simulink model "randomStuff"  (R2025a)
settings: Solver=VariableStepAuto  StartTime=0.0  StopTime=10.0  RelTol=1e-3
settings Model: Creator=willager  LastModifiedBy=willager

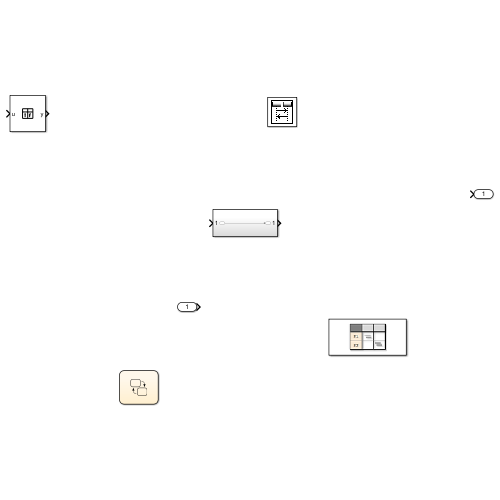
[thumbnail: Simulink's stored preview of the top-level diagram]
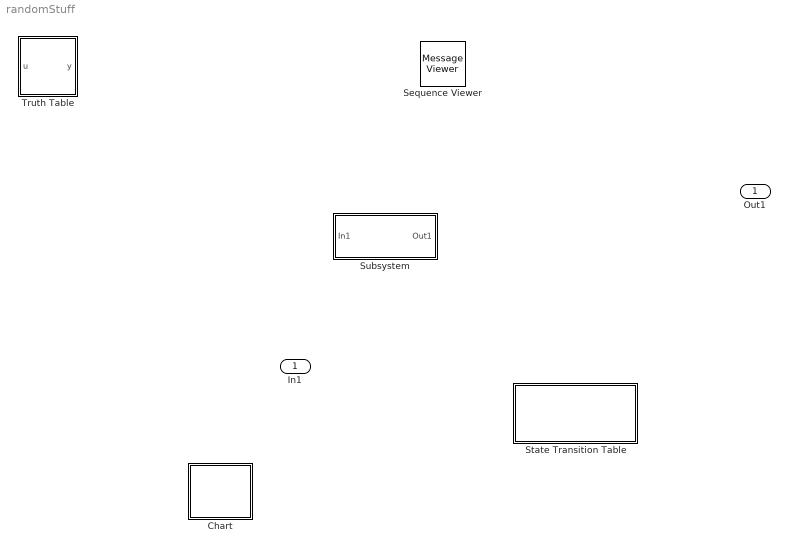
== system randomStuff ==
  In1 : Inport
  Chart : Stateflow chart  TreatAsAtomicUnit=on
  Sequence Viewer : MessageViewer
  State Transition Table : State Transition Table  TreatAsAtomicUnit=on
  Subsystem : Subsystem
  Truth Table : Truth Table  TreatAsAtomicUnit=on
  Out1 : Outport

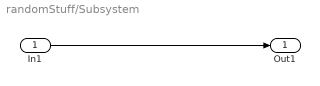
== system randomStuff/Subsystem ==
  In1 : Inport
  Out1 : Outport
  wires:
  In1/1 -> Out1/1

== matlab function randomStuff/Truth Table ==
  data: u input; y output
function y = fcn(u)

aVarTruthTableCondition_1 = false;
aVarTruthTableCondition_2 = false;


% Example condition 1

aVarTruthTableCondition_1 = logical(u >= 0);

% Example condition 2

aVarTruthTableCondition_2 = logical(u ^ 2 <= 1);

if (aVarTruthTableCondition_1 && aVarTruthTableCondition_2)
    aFcnTruthTableAction_1();
elseif (~aVarTruthTableCondition_1 && ~aVarTruthTableCondition_2)
    aFcnTruthTableAction_1();
else % Default
    aFcnTruthTableAction_2();
end

function aFcnTruthTableAction_1()

% Example action 1 called from D1 & D2 column in condition table

y = u;

function aFcnTruthTableAction_2()

% Example action 2 called from D3 column in condition table

y = 1 / u;

== stateflow chart randomStuff/Chart ==

== stateflow chart randomStuff/State Transition Table ==
  state state1
  state state2
  (default) -> state1
  state1 -> state2
